simulink model "Cruise_Control"  (R2020b)
settings: Solver=ode45  StartTime=0.0  StopTime=10  RelTol=1e-3
values from neighbouring files (symbols this model uses):
  b = 50.0    [data_dict.sldd]
  ki = 40.0    [data_dict.sldd]
  kp = 1000.0    [data_dict.sldd]
  m = 1000.0    [data_dict.sldd]
settings Model: DataDictionary=data_dict.sldd  Creator=Shree  LastModifiedBy=Shree

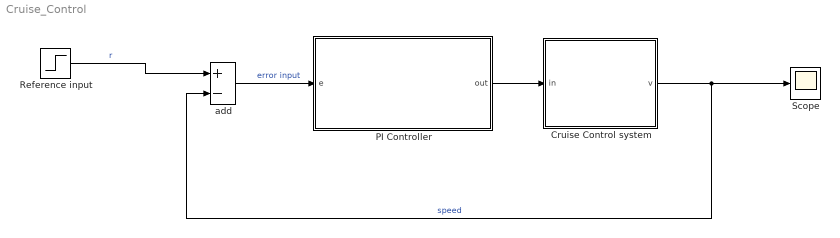
== system Cruise_Control ==
  Cruise Control system : Subsystem
  PI Controller : Subsystem
  Reference input : Step  Time=0  After=u  SampleTime=0
  Scope : Scope
  add : Sum  Inputs=+-
  wires:
  PI Controller/1(out) -> Cruise Control system/1(in)
  add/1 -> PI Controller/1(e)  "error input"
  Reference input/1 -> add/1  "r"
  Cruise Control system/1(v) -> Scope/1, add/2  "speed"

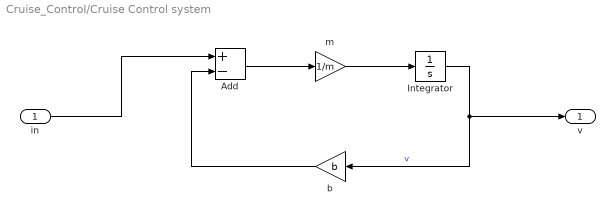
== system Cruise_Control/Cruise Control system ==
  in : Inport
  Add : Sum  Inputs=+-
  Integrator : Integrator
  b : Gain  Gain=b
  m : Gain  Gain=1/m
  v : Outport
  wires:
  in/1 -> Add/1
  Integrator/1 -> v/1, b/1  "v"
  b/1 -> Add/2
  m/1 -> Integrator/1
  Add/1 -> m/1

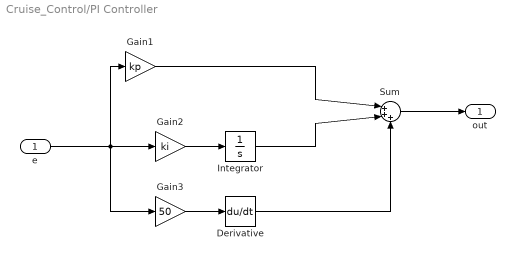
== system Cruise_Control/PI Controller ==
  e : Inport
  Derivative : Derivative
  Gain1 : Gain  Gain=kp
  Gain2 : Gain  Gain=ki
  Gain3 : Gain  Gain=50
  Integrator : Integrator
  Sum : Sum  Inputs=|+++
  out : Outport
  wires:
  Gain2/1 -> Integrator/1
  Integrator/1 -> Sum/2
  Sum/1 -> out/1
  Gain1/1 -> Sum/1
  e/1 -> Gain3/1, Gain1/1, Gain2/1
  Gain3/1 -> Derivative/1
  Derivative/1 -> Sum/3
